simulink library "neuromorphic_blocks"  (R2022a)
settings: Solver=VariableStepAuto  StartTime=0.0  StopTime=10.0  RelTol=1e-3
libraries: $bdroot x47, simulink x7
(part 3 of 3)

== system neuromorphic_blocks/Tunable Sigmoid/Sigmoid ==
  x : Inport
  Constant : Constant
  Gain : Gain  Gain=2
  Gain1 : Gain  Gain=0.5
  Sum : Sum  Inputs=|++
  Trigonometric Function : Trigonometry  Operator=tanh
  y : Outport
  wires:
  Gain/1 -> Trigonometric Function/1
  x/1 -> Gain/1
  Trigonometric Function/1 -> Sum/1
  Constant/1 -> Sum/2
  Sum/1 -> Gain1/1
  Gain1/1 -> y/1

== system neuromorphic_blocks/Auxiliary Blocks/Event-Signal Multiplier/VSub ==
  in : Inport
  s : Inport  Port=2
  Events : Subsystem  VariantControl=Events
  Voltage : Subsystem  VariantControl=Voltage
  out+ : Outport
  out- : Outport  Port=2

== system neuromorphic_blocks/Auxiliary Blocks/Event-Signal Selector/VSub ==
  in+ : Inport
  in- : Inport  Port=2
  s : Inport  Port=3
  Events : Subsystem  VariantControl=Events
  Voltage : Subsystem  VariantControl=Voltage
  out : Outport

== system neuromorphic_blocks/Events Transmission Blocks/Event Loss/Generate Random Number on Positive ==
  Trigger : TriggerPort  TriggerType=either  VariantControl=(inherit)  ShowOutputPort=on
  Constant : Constant  Value=0
  Switch : Switch  SaturateOnIntegerOverflow=off  InputSameDT=off
  Uniform Random Number1 : UniformRandomNumber  Minimum=0  Seed=seed_mem
  Out1 : Outport
  wires:
  Constant/1 -> Switch/3
  Trigger/1 -> Switch/2
  Uniform Random Number1/1 -> Switch/1
  Switch/1 -> Out1/1

== system neuromorphic_blocks/Events Transmission Blocks/Event to Fixed Width Pulse/Triggered Subsystem ==
  In1 : Inport
  Trigger : TriggerPort  VariantControl=(inherit)  InitialTriggerSignalState=zero
  Out1 : Outport  InitialOutput=-pulse_width
  wires:
  In1/1 -> Out1/1

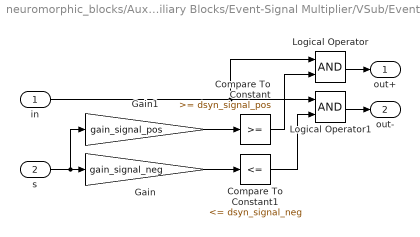
== system neuromorphic_blocks/Auxiliary Blocks/Event-Signal Multiplier/VSub/Events ==
  in : Inport
  s : Inport  Port=2
  Compare To Constant : simulink/Logic and Bit Operations/Compare To Constant  relop=>=  const=dsyn_signal_pos  OutDataTypeStr=boolean
  Compare To Constant1 : simulink/Logic and Bit Operations/Compare To Constant  relop=<=  const=dsyn_signal_neg  OutDataTypeStr=boolean
  Gain : Gain  Gain=gain_signal_neg
  Gain1 : Gain  Gain=gain_signal_pos
  Logical Operator : Logic  AllPortsSameDT=off  OutDataTypeStr=boolean
  Logical Operator1 : Logic  AllPortsSameDT=off  OutDataTypeStr=boolean
  out+ : Outport
  out- : Outport  Port=2
  wires:
  Compare To Constant/1 -> Logical Operator/2
  Compare To Constant1/1 -> Logical Operator1/2
  in/1 -> Logical Operator/1, Logical Operator1/1
  Logical Operator1/1 -> out-/1
  Logical Operator/1 -> out+/1
  s/1 -> Gain1/1, Gain/1
  Gain/1 -> Compare To Constant1/1
  Gain1/1 -> Compare To Constant/1

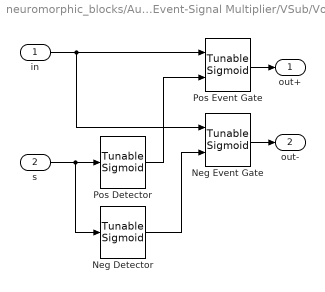
== system neuromorphic_blocks/Auxiliary Blocks/Event-Signal Multiplier/VSub/Voltage ==
  in : Inport
  s : Inport  Port=2
  Neg Detector : $bdroot/Tunable Sigmoid  nonlinearity_type=Sigmoid  gain_source=Internal  gain=gsyn_neg  bias=-dsyn_signal_neg  slope=-gain_signal_neg
  Neg Event Gate : $bdroot/Tunable Sigmoid  nonlinearity_type=Sigmoid  gain_source=External  gain=0  bias=dsyn_event_neg  slope=gain_event_neg
  Pos Detector : $bdroot/Tunable Sigmoid  nonlinearity_type=Sigmoid  gain_source=Internal  gain=gsyn_pos  bias=dsyn_signal_pos  slope=gain_signal_pos
  Pos Event Gate : $bdroot/Tunable Sigmoid  nonlinearity_type=Sigmoid  gain_source=External  gain=0  bias=dsyn_event_pos  slope=gain_event_pos
  out+ : Outport
  out- : Outport  Port=2
  wires:
  Neg Detector/1 -> Neg Event Gate/2
  in/1 -> Pos Event Gate/1, Neg Event Gate/1
  s/1 -> Neg Detector/1, Pos Detector/1
  Pos Detector/1 -> Pos Event Gate/2
  Pos Event Gate/1 -> out+/1
  Neg Event Gate/1 -> out-/1

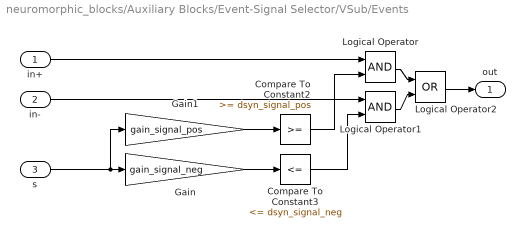
== system neuromorphic_blocks/Auxiliary Blocks/Event-Signal Selector/VSub/Events ==
  in+ : Inport
  in- : Inport  Port=2
  s : Inport  Port=3
  Compare To Constant2 : simulink/Logic and Bit Operations/Compare To Constant  relop=>=  const=dsyn_signal_pos  OutDataTypeStr=boolean
  Compare To Constant3 : simulink/Logic and Bit Operations/Compare To Constant  relop=<=  const=dsyn_signal_neg  OutDataTypeStr=boolean
  Gain : Gain  Gain=gain_signal_neg
  Gain1 : Gain  Gain=gain_signal_pos
  Logical Operator : Logic  AllPortsSameDT=off  OutDataTypeStr=boolean
  Logical Operator1 : Logic  AllPortsSameDT=off  OutDataTypeStr=boolean
  Logical Operator2 : Logic  Operator=OR  AllPortsSameDT=off  OutDataTypeStr=boolean
  out : Outport
  wires:
  Compare To Constant2/1 -> Logical Operator/2
  Compare To Constant3/1 -> Logical Operator1/2
  in+/1 -> Logical Operator/1
  in-/1 -> Logical Operator1/1
  Logical Operator2/1 -> out/1
  Logical Operator1/1 -> Logical Operator2/2
  Logical Operator/1 -> Logical Operator2/1
  Gain1/1 -> Compare To Constant2/1
  s/1 -> Gain/1, Gain1/1
  Gain/1 -> Compare To Constant3/1

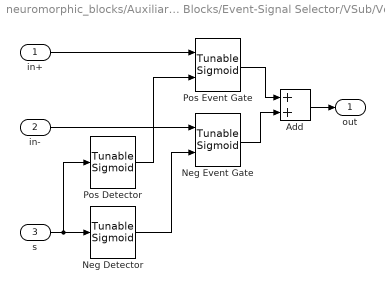
== system neuromorphic_blocks/Auxiliary Blocks/Event-Signal Selector/VSub/Voltage ==
  in+ : Inport
  in- : Inport  Port=2
  s : Inport  Port=3
  Add : Sum
  Neg Detector : $bdroot/Tunable Sigmoid  nonlinearity_type=Sigmoid  gain_source=Internal  gain=gsyn_neg  bias=-dsyn_signal_neg  slope=-gain_signal_neg
  Neg Event Gate : $bdroot/Tunable Sigmoid  nonlinearity_type=Sigmoid  gain_source=External  gain=0  bias=dsyn_event_neg  slope=gain_event_neg
  Pos Detector : $bdroot/Tunable Sigmoid  nonlinearity_type=Sigmoid  gain_source=Internal  gain=gsyn_pos  bias=dsyn_signal_pos  slope=gain_signal_pos
  Pos Event Gate : $bdroot/Tunable Sigmoid  nonlinearity_type=Sigmoid  gain_source=External  gain=0  bias=dsyn_event_pos  slope=gain_event_pos
  out : Outport
  wires:
  Add/1 -> out/1
  Neg Event Gate/1 -> Add/2
  Pos Detector/1 -> Pos Event Gate/2
  in+/1 -> Pos Event Gate/1
  in-/1 -> Neg Event Gate/1
  Pos Event Gate/1 -> Add/1
  Neg Detector/1 -> Neg Event Gate/2
  s/1 -> Neg Detector/1, Pos Detector/1
